simulink model "main_simulation_2018a"  (R2018a)
settings: Solver=VariableStepAuto  StartTime=0.0  StopTime=10.0  RelTol=1e-3
settings Model: Creator=rolka  LastModifiedBy=Emilian Rejman
settings DataIOCC: ReturnWorkspaceOutputs=on
settings SFSimCC: SimUseLocalCustomCode=on
settings RTWCC: RTWUseLocalCustomCode=on

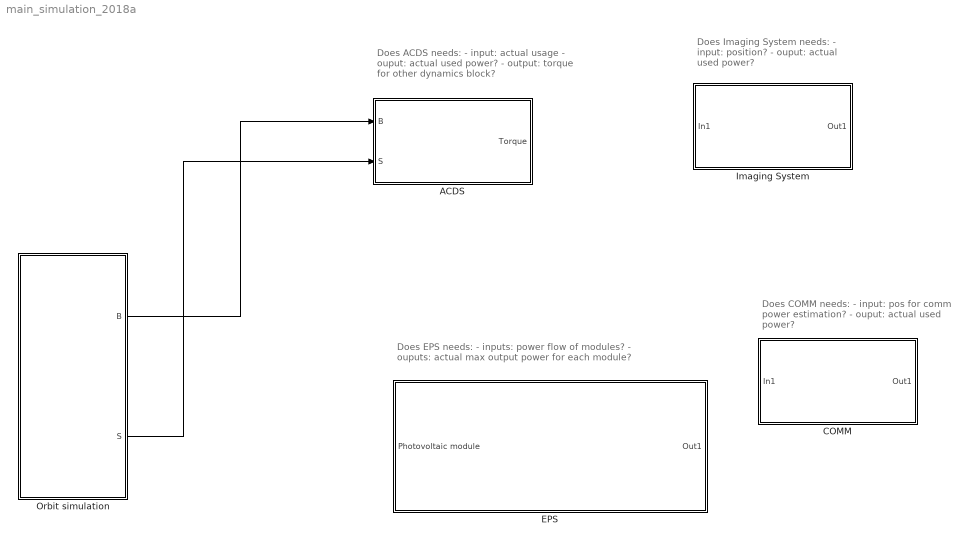
== system main_simulation_2018a ==
  note: Does Imaging System needs:
      | - input: position?
      | - ouput: actual used power?
  note: Does EPS needs:
      | - inputs: power flow of modules?
      | - ouputs: actual max output power for each module?
  note: Does COMM needs:
      | - input: pos for comm power estimation?
      | - ouput: actual used power?
  note: Does ACDS needs:
      | - input: actual usage
      | - ouput: actual used power?
      | - output: torque for other dynamics block?
  ACDS : Subsystem
  COMM : Subsystem
  EPS : Subsystem
  Imaging System : Subsystem
  Orbit simulation : Subsystem
  wires:
  Orbit simulation/1(B) -> ACDS/1(B)
  Orbit simulation/2(S) -> ACDS/2(S)

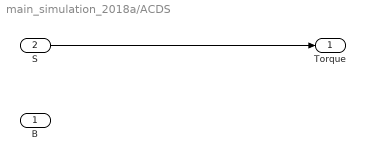
== system main_simulation_2018a/ACDS ==
  B : Inport
  S : Inport  Port=2
  Torque : Outport  VectorParamsAs1DForOutWhenUnconnected=on
  wires:
  S/1 -> Torque/1

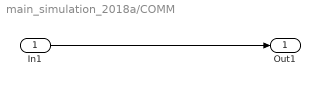
== system main_simulation_2018a/COMM ==
  In1 : Inport
  Out1 : Outport  VectorParamsAs1DForOutWhenUnconnected=on
  wires:
  In1/1 -> Out1/1

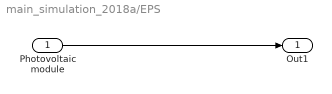
== system main_simulation_2018a/EPS ==
  Photovoltaic module : Inport
  Out1 : Outport  VectorParamsAs1DForOutWhenUnconnected=on
  wires:
  Photovoltaic module/1 -> Out1/1

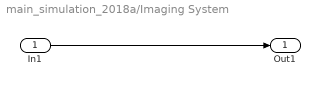
== system main_simulation_2018a/Imaging System ==
  In1 : Inport
  Out1 : Outport  VectorParamsAs1DForOutWhenUnconnected=on
  wires:
  In1/1 -> Out1/1

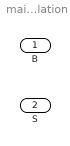
== system main_simulation_2018a/Orbit simulation ==
  B : Outport  VectorParamsAs1DForOutWhenUnconnected=on
  S : Outport  Port=2  VectorParamsAs1DForOutWhenUnconnected=on
